simulink library "asbCubeSatFSWLib"  (R2023a)
settings: Solver=VariableStepAuto  StartTime=0.0  StopTime=10.0  RelTol=1e-3
settings Model: Creator=The MathWorks, Inc.  LastModifiedBy=The MathWorks, Inc.
settings SolverCC: AlgebraicLoopSolver=TrustRegion  MaxZcPerStep=1
settings DebuggingCC: UnconnectedInputMsg=warning  UnconnectedOutputMsg=warning  UnconnectedLineMsg=warning
settings ModelReferenceCC: EnableRefExpFcnMdlSchedulingChecks=on

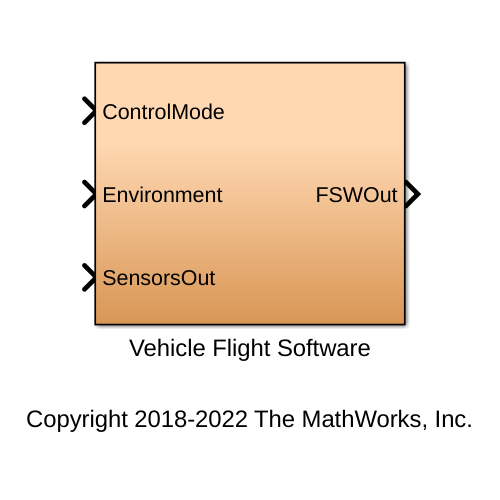
[thumbnail: Simulink's stored preview of the top-level diagram]
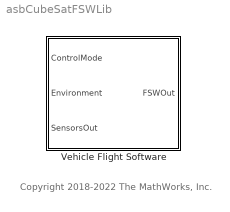
== system asbCubeSatFSWLib ==
  note: Copyright 2018-2022 The MathWorks, Inc.
  Vehicle Flight Software : Subsystem

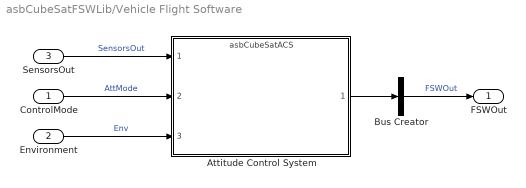
== system asbCubeSatFSWLib/Vehicle Flight Software ==
  ControlMode : Inport
  Environment : Inport  Port=2
  SensorsOut : Inport  Port=3  OutDataTypeStr=Bus: StatesOutBus
  Attitude Control System : ModelReference  ModelNameDialog=asbCubeSatACS.slx  SimulationMode=Normal  ModelReferenceVersion=7.0
  Bus Creator : BusCreator  Inputs=1  OutDataTypeStr=Bus: FCSOutBus  NonVirtualBus=on
  FSWOut : Outport  OutDataTypeStr=Bus: FCSOutBus  VectorParamsAs1DForOutWhenUnconnected=off
  wires:
  Bus Creator/1 -> FSWOut/1  "FSWOut"
  Attitude Control System/1 -> Bus Creator/1
  ControlMode/1 -> Attitude Control System/2  "AttMode"
  SensorsOut/1 -> Attitude Control System/1  "SensorsOut"
  Environment/1 -> Attitude Control System/3  "Env"
